simulink model "modelGod"  (Simulink 10.2)
settings: Solver=FixedStepAuto  StartTime=0.0  StopTime=200  FixedStep=0.001  MaxStep=0.01  RelTol=1e-3
values from neighbouring files (symbols this model uses):
  A = [-Ya_Alpha 1 0 ... (first row only)    [StateSpace.m]    (also in matan.m = [1 -1/p; modelGodPrint.m = figure; print2.m = figure)
  B = [0;Mz_deltaB;0]    [StateSpace.m]    (also in matan.m = [0; -K_v*Vzad/(1/(W*Wpriv)+K_wz)]; modelGodPrint.m = figure)
  C = [1 0 0; 0 1 0; 0 0 1]    [StateSpace.m]    (also in modelGodPrint.m = figure)
  D = [0;0;0]    [StateSpace.m]    (also in modelGodPrint.m = figure)
  i_H = 0.8/(1/Ya_Alpha*V)    [Synthesis_of_ACS.m]
  i_p = i_H^2*V    [Synthesis_of_ACS.m]
  K_v = nu*K_wz    [Synthesis_of_ACS.m]
  K_wz = e*K_wzGr    [Synthesis_of_ACS.m]
  w = max(w1)    [DriveParameters.m]
settings Model: Creator=User  LastModifiedBy=User
settings DataIOCC: SaveFormat=Dataset  SignalLoggingSaveFormat=Dataset  ReturnWorkspaceOutputs=on
settings OptimizationCC: LifeSpan=auto
settings DebuggingCC: UnderspecifiedInitializationDetection=Simplified  MergeDetectMultiDrivingBlocksExec=error  FcnCallInpInsideContextMsg=error  SFUnexpectedBacktrackingDiag=error  SFNoUnconditionalDefaultTransitionDiag=error  SFExecutionAtInitializationDiag=warning  ArithmeticOperatorsInVariantConditions=error
settings HardwareCC: ProdBitPerPointer=64  ProdBitPerSizeT=64  ProdBitPerPtrDiffT=64  ProdLargestAtomicFloat=Float  ProdIntDivRoundTo=Zero  ProdEndianess=LittleEndian  ProdWordSize=64  ProdHWDeviceType=Intel->x86-64 (Windows64)
settings ModelReferenceCC: PropagateSignalLabelsOutOfModel=on
settings SFSimCC: SimUseLocalCustomCode=on
settings RTWCC: RTWUseLocalCustomCode=on
settings CodeAppCC: StateflowObjectComments=off
settings GRTTargetCC: TargetLangStandard=C99 (ISO)  CombineOutputUpdateFcns=on  GRTInterface=off
settings ConfigComp: CovMetricSettings=dwe  CovSaveCumulativeToWorkspaceVar=off  CovSaveSingleToWorkspaceVar=off  CovExternalEMLEnable=on

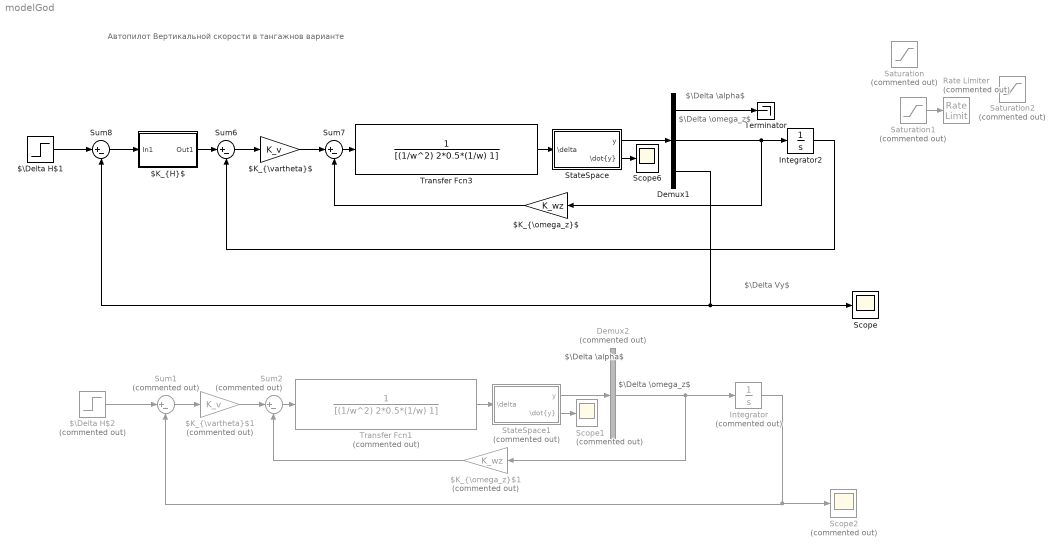
== system modelGod ==
  note: Автопилот Вертикальной скорости в тангажнов варианте
  note: $\Delta Vy$
  note: $\Delta \omega_z$
  note: $\Delta \alpha$
  note: $\Delta \alpha$
  note: $\Delta \omega_z$
  "$K_{H}$" : Subsystem
  "$K_{\\omega_z}$" : Gain  Gain=K_wz
  "$K_{\\omega_z}$1" : Gain  Commented=on  Gain=K_wz
  "$K_{\\vartheta}$" : Gain  Gain=K_v
  "$K_{\\vartheta}$1" : Gain  Commented=on  Gain=K_v
  $\Delta H$1 : Step  SampleTime=0
  $\Delta H$2 : Step  Commented=on  SampleTime=0
  Demux1 : Demux  Outputs=3
  Demux2 : Demux  Commented=on  Outputs=3
  Integrator : Integrator  Commented=on
  Integrator2 : Integrator
  Rate Limiter : RateLimiter  Commented=on  RisingSlewLimit=15*pi/180  FallingSlewLimit=-15*pi/180  SampleTimeMode=inherited
  Saturation : Saturate  Commented=on  UpperLimit=9*pi/180  LowerLimit=-9*pi/180
  Saturation1 : Saturate  Commented=on  UpperLimit=30*pi/180  LowerLimit=-30*pi/180
  Saturation2 : Saturate  Commented=on  UpperLimit=5*pi/180/0.001  LowerLimit=-5*pi/180/0.001
  Scope : Scope
  Scope1 : Scope  Commented=on
  Scope2 : Scope  Commented=on
  Scope6 : Scope
  StateSpace : Subsystem
  StateSpace1 : Subsystem  Commented=on
  Sum1 : Sum  Commented=on  Inputs=|+-
  Sum2 : Sum  Commented=on  Inputs=|+-
  Sum6 : Sum  Inputs=|+-
  Sum7 : Sum  Inputs=|+-
  Sum8 : Sum  Inputs=|+-
  Terminator : Terminator
  Transfer Fcn1 : TransferFcn  Commented=on  Denominator=[(1/w^2) 2*0.5*(1/w) 1]
  Transfer Fcn3 : TransferFcn  Denominator=[(1/w^2) 2*0.5*(1/w) 1]
  wires:
  "$K_{\\vartheta}$"/1 -> Sum7/1
  StateSpace/2("\\dot{y}") -> Scope6/1
  Demux1/2 -> Integrator2/1, "$K_{\\omega_z}$"/1
  StateSpace/1(y) -> Demux1/1
  Sum6/1 -> "$K_{\\vartheta}$"/1
  "$K_{H}$"/1(Out1) -> Sum6/1
  Saturation1/1 -> Rate Limiter/1
  $\Delta H$1/1 -> Sum8/1
  Sum8/1 -> "$K_{H}$"/1(In1)
  Sum7/1 -> Transfer Fcn3/1
  Transfer Fcn3/1 -> StateSpace/1(\delta)
  "$K_{\\omega_z}$"/1 -> Sum7/2
  Integrator2/1 -> Sum6/2
  Demux1/3 -> Scope/1, Sum8/2
  Demux1/1 -> Terminator/1
  Sum2/1 -> Transfer Fcn1/1
  "$K_{\\omega_z}$1"/1 -> Sum2/2
  Transfer Fcn1/1 -> StateSpace1/1(\delta)
  Sum1/1 -> "$K_{\\vartheta}$1"/1
  StateSpace1/2("\\dot{y}") -> Scope1/1
  "$K_{\\vartheta}$1"/1 -> Sum2/1
  Demux2/2 -> "$K_{\\omega_z}$1"/1, Integrator/1
  $\Delta H$2/1 -> Sum1/1
  StateSpace1/1(y) -> Demux2/1
  Integrator/1 -> Scope2/1, Sum1/2

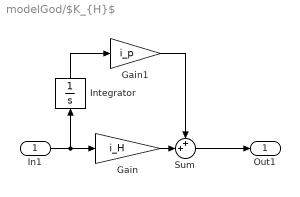
== system modelGod/$K_{H}$ ==
  In1 : Inport
  Gain : Gain  Gain=i_H
  Gain1 : Gain  Gain=i_p
  Integrator : Integrator
  Sum : Sum  Inputs=++|
  Out1 : Outport
  wires:
  Sum/1 -> Out1/1
  In1/1 -> Integrator/1, Gain/1
  Integrator/1 -> Gain1/1
  Gain/1 -> Sum/2
  Gain1/1 -> Sum/1

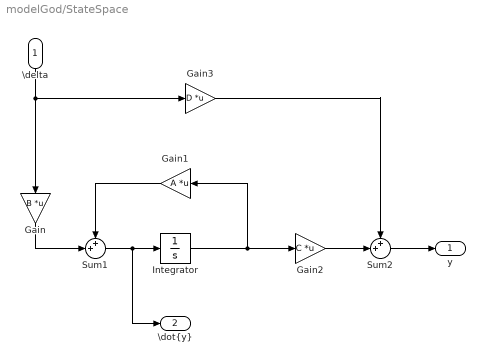
== system modelGod/StateSpace ==
  \delta : Inport
  Gain : Gain  Gain=B  Multiplication=Matrix(K*u)
  Gain1 : Gain  Gain=A  Multiplication=Matrix(K*u)
  Gain2 : Gain  Gain=C  Multiplication=Matrix(K*u)
  Gain3 : Gain  Gain=D  Multiplication=Matrix(K*u)
  Integrator : Integrator
  Sum1 : Sum  Inputs=++|
  Sum2 : Sum  Inputs=++|
  y : Outport
  "\\dot{y}" : Outport  Port=2
  wires:
  \delta/1 -> Gain/1, Gain3/1
  Sum1/1 -> "\\dot{y}"/1, Integrator/1
  Gain/1 -> Sum1/2
  Integrator/1 -> Gain2/1, Gain1/1
  Gain1/1 -> Sum1/1
  Gain2/1 -> Sum2/2
  Sum2/1 -> y/1
  Gain3/1 -> Sum2/1

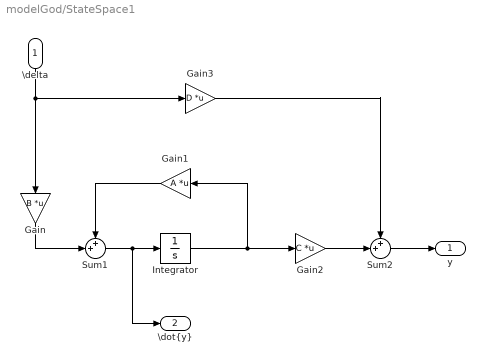
== system modelGod/StateSpace1 ==
  \delta : Inport
  Gain : Gain  Gain=B  Multiplication=Matrix(K*u)
  Gain1 : Gain  Gain=A  Multiplication=Matrix(K*u)
  Gain2 : Gain  Gain=C  Multiplication=Matrix(K*u)
  Gain3 : Gain  Gain=D  Multiplication=Matrix(K*u)
  Integrator : Integrator
  Sum1 : Sum  Inputs=++|
  Sum2 : Sum  Inputs=++|
  y : Outport
  "\\dot{y}" : Outport  Port=2
  wires:
  \delta/1 -> Gain/1, Gain3/1
  Sum1/1 -> "\\dot{y}"/1, Integrator/1
  Gain/1 -> Sum1/2
  Integrator/1 -> Gain2/1, Gain1/1
  Gain1/1 -> Sum1/1
  Gain2/1 -> Sum2/2
  Sum2/1 -> y/1
  Gain3/1 -> Sum2/1
